simulink model "Selector_TestGen16"  (R2017b)
settings: Solver=FixedStepDiscrete  StartTime=0.0  StopTime=10.0  RelTol=1e-3
undefined symbols (not defined in the file): Block_TestLib, enable_trigger
settings Model: Creator=ktrinh  LastModifiedBy=ktrinh
settings DebuggingCC: ParameterOverflowMsg=none

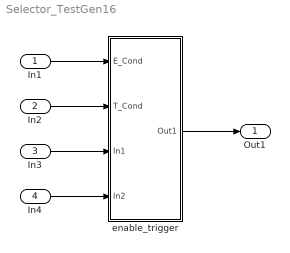
== system Selector_TestGen16 ==
  In1 : Inport
  In2 : Inport  Port=2
  In3 : Inport  Port=3
  In4 : Inport  Port=4
  enable_trigger : Subsystem  AncestorBlock=Block_TestLib/enable_trigger
  Out1 : Outport
  wires:
  In1/1 -> enable_trigger/1(E_Cond)
  In2/1 -> enable_trigger/2(T_Cond)
  In3/1 -> enable_trigger/3(In1)
  In4/1 -> enable_trigger/4(In2)
  enable_trigger/1(Out1) -> Out1/1

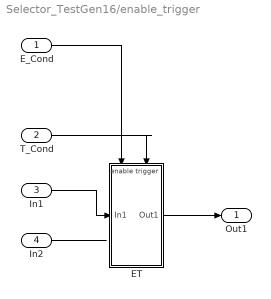
== system Selector_TestGen16/enable_trigger ==
  E_Cond : Inport  OutDataTypeStr=boolean
  T_Cond : Inport  Port=2  OutDataTypeStr=boolean
  In1 : Inport  Port=3
  In2 : Inport  Port=4
  ET : Subsystem  TreatAsAtomicUnit=on
  Out1 : Outport
  wires:
  T_Cond/1 -> ET/Trigger
  E_Cond/1 -> ET/Enable
  In1/1 -> ET/1(In1)
  In2/1 -> ?
  ET/1(Out1) -> Out1/1

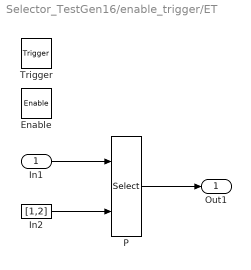
== system Selector_TestGen16/enable_trigger/ET ==
  In1 : Inport  OutDataTypeStr=double  PortDimensions=[3 2 2 2]
  Enable : EnablePort
  Trigger : TriggerPort  VariantControl=Variant
  In2 : Constant  Value=[1,2]
  P : Selector  NumberOfDimensions=4  InputPortWidth=3  IndexOptions=Select all,Index vector (dialog),Index vector (port),Starting index (dialog)  Indices=[],[1,2],[],1  OutputSizes=,,,2
  Out1 : Outport
  wires:
  In1/1 -> P/1
  In2/1 -> P/2
  P/1 -> Out1/1
